simulink model "can_model"  (R2026a)
settings: Solver=VariableStepAuto  StopTime=100
undefined symbols (not defined in the file): canChannel
libraries: canlib x5, canmsglib x4
settings Model: Creator=Giuseppe Grano  LastModifiedBy=Giuseppe Grano
settings SFSimCC: SimCustomHeaderCode=framework.h  SimUserIncludeDirs=.\Ascon
settings SFSimCC: SimUserSources=|
  | framework.c
  | .\Ascon\encrypt.c .\Ascon\core.c .\Ascon\permutations.c .\Ascon\decrypt.c

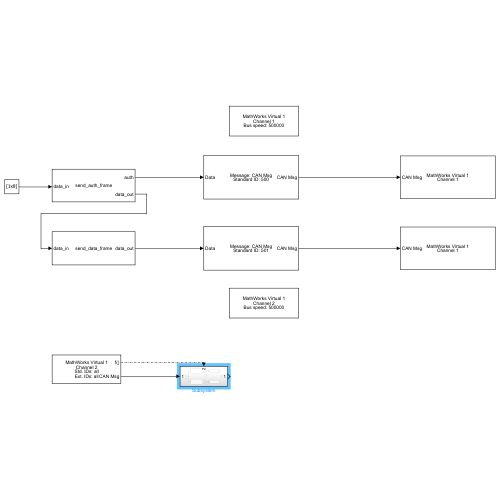
[thumbnail: Simulink's stored preview of the top-level diagram]
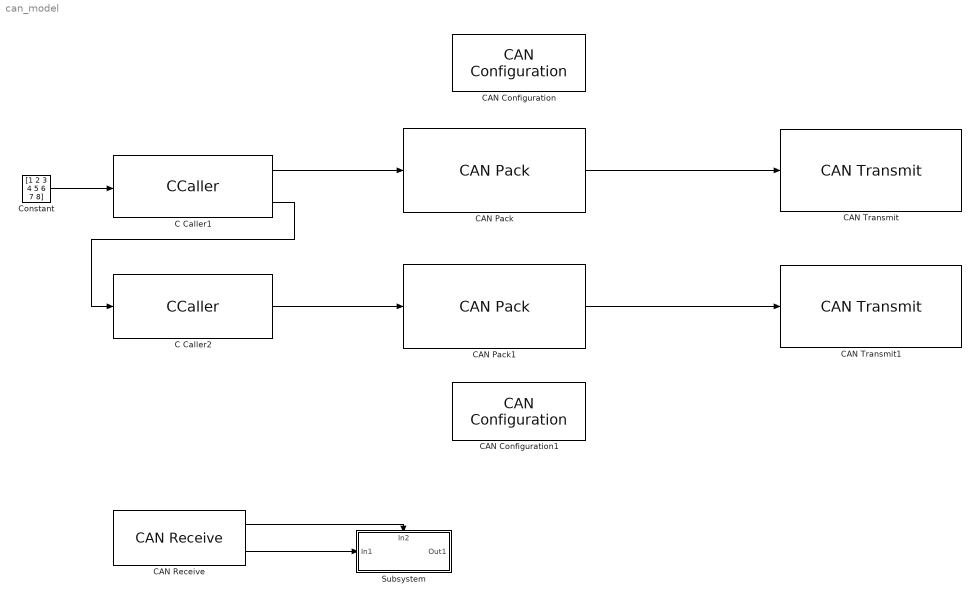
== system can_model ==
  C Caller1 : CCaller  FunctionName=send_auth_frame  PortSpecificationStruct="%)30     .    > 4   8    (     @         %    \"     ,    !     0         %  0 \"0    $    _    07)G3F%M90  4&]R=$YA;64 4V-O<&4     26YD97@     5'EP90      4VEZ90      27-';&]B86P   X    X    !@    @    $          4    (     0    <    !         !     '    9&%T85]I;@ .    .     8    (    !          %    \"     $    '     0         0    !P   &1A=&%?:6X #@   #@    &    \"     0         !0    @    !    !0    $         $     4   !);G!U=     X    X    !@    @    &          4    (     0    $    !          D    (               .    .     8    (    !          %    \"     $    %     0         0    !0   '5I;G0X    #@   #     &    \"     0         !0    @    !     0    $         $  ! #@    .    ,     8    (    \"0(        %    \"     $    !     0         \"  $       X    P    !@    @    $          4    (     0    0    !         !  ! !A=71H#@   #     &    \"     0         !0    @    !    !     $         $  $ &%U=&@.    .     8    (    !          %    \"     $    &     0         0    !@   $]U='!U=   #@   #@    &    \"     8         !0    @    !     0    $         \"0    @               X    X    !@    @    $          4    (     0    4    !         !     %    =6EN=#@    .    ,     8    (    !          %    \"     $    !     0         0  $ .     X    P    !@    @    ) @        4    (     0    $    !          (  0      #@   #@    &    \"     0         !0    @    !    \"     $         $     @   !D871A7V]U= X    X    !@    @    $          4    (     0    @    !         !     (    9&%T85]O=70.    .     8    (    !          %    \"     $    &     0         0    !@   $]U='!U=   #@   #@    &    \"     8         !0    @    !     0    $         \"0    @           #P/PX    X    !@    @    $          4    (     0    4    !         !     %    =6EN=#@    .    ,     8    (    !          %    \"     $    !     0         0  $ .     X    P    !@    @    ) @        4    (     0    $    !          (  0"
  C Caller2 : CCaller  FunctionName=send_data_frame  PortSpecificationStruct="%)30     .    V ,   8    (     @         %    \"     (    !     0         %  0 \"0    $    _    07)G3F%M90  4&]R=$YA;64 4V-O<&4     26YD97@     5'EP90      4VEZ90      27-';&]B86P   X    X    !@    @    $          4    (     0    <    !         !     '    9&%T85]I;@ .    .     8    (    !          %    \"     $    '     0         0    !P   &1A=&%?:6X #@   #@    &    \"     0         !0    @    !    !0    $         $     4   !);G!U=     X    X    !@    @    &          4    (     0    $    !          D    (               .    .     8    (    !          %    \"     $    %     0         0    !0   '5I;G0X    #@   #     &    \"     0         !0    @    !     0    $         $  ! #@    .    ,     8    (    \"0(        %    \"     $    !     0         \"  $       X    X    !@    @    $          4    (     0    @    !         !     (    9&%T85]O=70.    .     8    (    !          %    \"     $    (     0         0    \"    &1A=&%?;W5T#@   #@    &    \"     0         !0    @    !    !@    $         $     8   !/=71P=70   X    X    !@    @    &          4    (     0    $    !          D    (               .    .     8    (    !          %    \"     $    %     0         0    !0   '5I;G0X    #@   #     &    \"     0         !0    @    !     0    $         $  ! #@    .    ,     8    (    \"0(        %    \"     $    !     0         \"  $"
  CAN Configuration : canlib/CAN Configuration  BlockHandle=160.0001  Device=MathWorks Virtual 1 (Channel 1)  DeviceMenu=MathWorks Virtual 1 (Channel 1)  ObjConstructor=canChannel('MathWorks', 'Virtual 1', 1)  BusSpeed=500000  EnableBitParameters=off  AckMode=Normal
  CAN Configuration1 : canlib/CAN Configuration  BlockHandle=161.0001  Device=MathWorks Virtual 1 (Channel 2)  DeviceMenu=MathWorks Virtual 1 (Channel 2)  ObjConstructor=canChannel('MathWorks', 'Virtual 1', 2)  BusSpeed=500000  EnableBitParameters=off  AckMode=Normal
  CAN Pack : canmsglib/CAN Pack  MsgList=(none)  MsgName=CAN Msg  MsgIDType=Standard (11-bit identifier)  MsgIdentifier=500  CANIDInput=off  MsgLength=8  Remote=off  ApplyMinMax=off  BusOutput=off  SignalInfo={}
      settings: LibrarySourceBlock=canlib/CAN Pack  DataFormat=raw data
  CAN Pack1 : canmsglib/CAN Pack  MsgList=(none)  MsgName=CAN Msg  MsgIDType=Standard (11-bit identifier)  MsgIdentifier=501  CANIDInput=off  MsgLength=8  Remote=off  ApplyMinMax=off  BusOutput=off  SignalInfo={}
      settings: LibrarySourceBlock=canlib/CAN Pack  DataFormat=raw data
  CAN Receive : canlib/CAN Receive  BlockHandle=168.0001  Device=MathWorks Virtual 1 (Channel 2)  DeviceMenu=MathWorks Virtual 1 (Channel 2)  ObjConstructor=canChannel('MathWorks', 'Virtual 1', 2)  EnableStandardIDsFilter=off  StdIDsCombo=Allow all  StandardIDs=0  EnableExtendedIDsFilter=off  ExtIDsCombo=Allow all  ExtendedIDs=0  SampleTime=0.005  MsgsPerTimestep=1  InternalFilterUpdateStatus=on  BusOutput=off
  CAN Transmit : canlib/CAN Transmit  BlockHandle=171.0001  Device=MathWorks Virtual 1 (Channel 1)  DeviceMenu=MathWorks Virtual 1 (Channel 1)  ObjConstructor=canChannel('MathWorks', 'Virtual 1', 1)  EnableEventTransmit=off  EnablePeriodicTransmit=off  MessagePeriod=1.000
  CAN Transmit1 : canlib/CAN Transmit  BlockHandle=173.0001  Device=MathWorks Virtual 1 (Channel 1)  DeviceMenu=MathWorks Virtual 1 (Channel 1)  ObjConstructor=canChannel('MathWorks', 'Virtual 1', 1)  EnableEventTransmit=off  EnablePeriodicTransmit=off  MessagePeriod=1.000
  Constant : Constant  Value=[1 2 3 4 5 6 7 8]  OutDataTypeStr=uint8  SampleTime=0.01
  Subsystem : Subsystem
      settings: PortSchema="{\"entries\":[{\"content\":{\"sides\":[{\"content\":{\"connectorIds\":[\"In1\"]},\"type\":\"ConnectorPlacement.EquallySpacedRectSide\",\"uuid\":\"9c9d8698-828c-459a-b541-2e3dd4c23405\"},{\"content\":{\"connectorIds\":[\"Out1\"],\"side\":\"RIGHT\"},\"type\":\"ConnectorPlacement.EquallySpacedRectSide\",\"uuid\":\"238bd8db-bfb2-41f4-bbb5-5584c20a78df\"},{\"content\":{\"connectorIds\":[\"In2\"],\"side\":\"TOP\"},\"type\":\"ConnectorPlacement.EquallySpacedRectSide\",\"uuid\":\"a63b7d63-907f-4b9c-ab39-ca6e086bf702\"}]},\"type\":\"ConnectorPlacement.EquallySpacedConnector\",\"uuid\":\"3c9bb4e8-afbd-4aa6-a6bc-d7b61b368d58\"}],\"packageUris\":[\"http://schema.mathworks.com/mf0/Connector/R2020b\"],\"version\":\"1.0\"}"
  wires:
  CAN Pack/1 -> CAN Transmit/1
  Constant/1 -> C Caller1/1
  C Caller1/1 -> CAN Pack/1
  C Caller1/2 -> C Caller2/1
  C Caller2/1 -> CAN Pack1/1
  CAN Pack1/1 -> CAN Transmit1/1
  CAN Receive/2 -> Subsystem/1(In1)
  CAN Receive/1 -> Subsystem/2(In2)

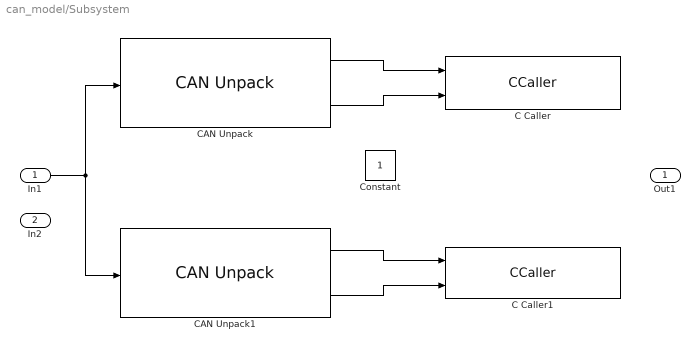
== system can_model/Subsystem ==
  In1 : Inport
  In2 : Inport  Port=2
  C Caller : CCaller  FunctionName=receive_auth_frame  PortSpecificationStruct="%)30     .    B 4   8    (     @         %    \"     ,    !     0         %  0 \"0    $    _    07)G3F%M90  4&]R=$YA;64 4V-O<&4     26YD97@     5'EP90      4VEZ90      27-';&]B86P   X    X    !@    @    $          4    (     0    8    !         !     &    ;7-G7VEN   .    .     8    (    !          %    \"     $    &     0         0    !@   &US9U]I;@  #@   #@    &    \"     0         !0    @    !    !0    $         $     4   !);G!U=     X    X    !@    @    &          4    (     0    $    !          D    (               .    .     8    (    !          %    \"     $    %     0         0    !0   '5I;G0X    #@   #     &    \"     0         !0    @    !     0    $         $  ! #@    .    ,     8    (    \"0(        %    \"     $    !     0         \"  $       X    X    !@    @    $          4    (     0    @    !         !     (    875T:%]O=70.    .     8    (    !          %    \"     $    (     0         0    \"    &%U=&A?;W5T#@   #@    &    \"     0         !0    @    !    !@    $         $     8   !/=71P=70   X    X    !@    @    &          4    (     0    $    !          D    (               .    .     8    (    !          %    \"     $    %     0         0    !0   '5I;G0X    #@   #     &    \"     0         !0    @    !     0    $         $  ! #$    .    ,     8    (    \"0(        %    \"     $    !     0         \"  $       X    X    !@    @    $          4    (     0    8    !         !     &    <W1A='5S   .    .     8    (    !          %    \"     $    &     0         0    !@   '-T871U<P  #@   #@    &    \"     0         !0    @    !    !0    $         $     4   !);G!U=     X    X    !@    @    &          4    (     0    $    !          D    (            \\#\\.    .     8    (    !          %    \"     $    %     0         0    !0   '5I;G0X    #@   #     &    \"     0         !0    @    !     0    $         $  ! #$    .    ,     8    (    \"0(        %    \"     $    !     0         \"  $"
  C Caller1 : CCaller  FunctionName=receive_data_frame  PortSpecificationStruct="%)30     .    V ,   8    (     @         %    \"     (    !     0         %  0 \"0    $    _    07)G3F%M90  4&]R=$YA;64 4V-O<&4     26YD97@     5'EP90      4VEZ90      27-';&]B86P   X    X    !@    @    $          4    (     0    8    !         !     &    ;7-G7VEN   .    .     8    (    !          %    \"     $    &     0         0    !@   &US9U]I;@  #@   #@    &    \"     0         !0    @    !    !0    $         $     4   !);G!U=     X    X    !@    @    &          4    (     0    $    !          D    (               .    .     8    (    !          %    \"     $    %     0         0    !0   '5I;G0X    #@   #     &    \"     0         !0    @    !     0    $         $  ! #@    .    ,     8    (    \"0(        %    \"     $    !     0         \"  $       X    X    !@    @    $          4    (     0    8    !         !     &    <W1A='5S   .    .     8    (    !          %    \"     $    &     0         0    !@   '-T871U<P  #@   #@    &    \"     0         !0    @    !    !0    $         $     4   !);G!U=     X    X    !@    @    &          4    (     0    $    !          D    (            \\#\\.    .     8    (    !          %    \"     $    %     0         0    !0   '5I;G0X    #@   #     &    \"     0         !0    @    !     0    $         $  ! #$    .    ,     8    (    \"0(        %    \"     $    !     0         \"  $"
  CAN Unpack : canmsglib/CAN Unpack  MsgList=(none)  MsgName=CAN Msg  MsgIDType=Standard (11-bit identifier)  MsgIdentifier=500  MsgLength=8  SignalInfo={}  IDPort=off  TimestampPort=off  ErrorPort=off  RemotePort=off  LengthPort=off  StatusPort=on  ApplyMinMax=off
      settings: LibrarySourceBlock=canlib/CAN Unpack  DataFormat=raw data
  CAN Unpack1 : canmsglib/CAN Unpack  MsgList=(none)  MsgName=CAN Msg  MsgIDType=Standard (11-bit identifier)  MsgIdentifier=501  MsgLength=8  SignalInfo={}  IDPort=off  TimestampPort=off  ErrorPort=off  RemotePort=off  LengthPort=off  StatusPort=on  ApplyMinMax=off
      settings: LibrarySourceBlock=canlib/CAN Unpack  DataFormat=raw data
  Constant : Constant  OutDataTypeStr=uint8
  Out1 : Outport
  wires:
  In1/1 -> CAN Unpack1/1, CAN Unpack/1
  CAN Unpack/1 -> C Caller/1
  CAN Unpack1/1 -> C Caller1/1
  CAN Unpack/2 -> C Caller/2
  CAN Unpack1/2 -> C Caller1/2
